simulink subsystem "SubsistemaMotor"  (R2022b)
settings: Solver=VariableStepAuto  StartTime=0.0  StopTime=10.0  RelTol=1e-3
libraries: arduinolib x6, simulink x2
settings Model: Creator=manu_  LastModifiedBy=manu_

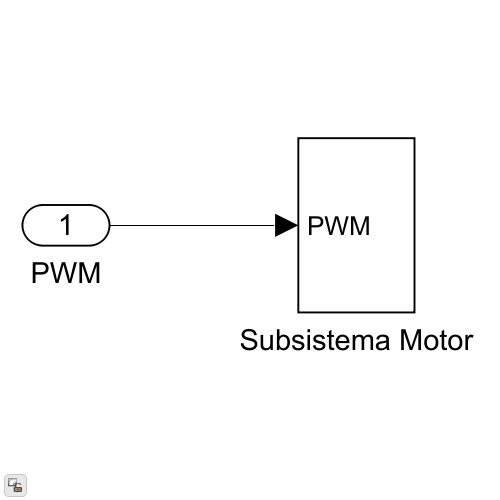
[thumbnail: Simulink's stored preview of the top-level diagram]
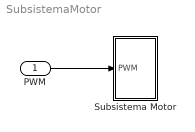
== system SubsistemaMotor ==
  PWM : Inport
  Subsistema Motor : Subsystem
  wires:
  PWM/1 -> Subsistema Motor/1(PWM)

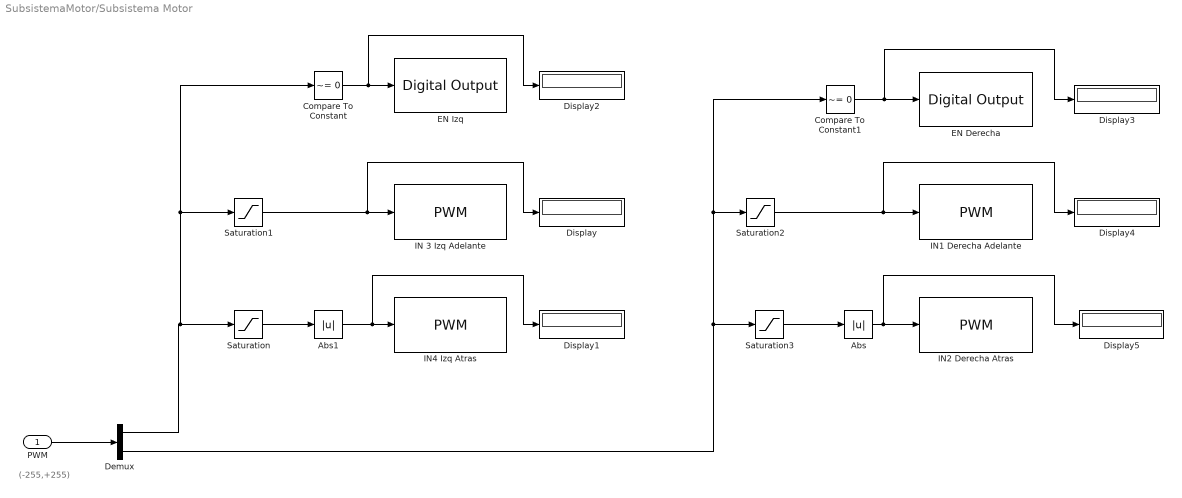
== system SubsistemaMotor/Subsistema Motor ==
  note: (-255,+255)
  PWM : Inport
  Abs : Abs  SaturateOnIntegerOverflow=off
  Abs1 : Abs  SaturateOnIntegerOverflow=off
  Compare To Constant : simulink/Logic and Bit Operations/Compare To Constant  relop=~=  const=0  OutDataTypeStr=boolean
  Compare To Constant1 : simulink/Logic and Bit Operations/Compare To Constant  relop=~=  const=0  OutDataTypeStr=boolean
  Demux : Demux  Outputs=2
  Display{,1..5} (6 alike) : Display
  EN Derecha : arduinolib/Digital Output  pinNumber=8  Direction=output  blockPlatform=arduino
  EN Izq : arduinolib/Digital Output  pinNumber=13  Direction=output  blockPlatform=arduino
  IN 3 Izq Adelante : arduinolib/PWM  pinNumber=11  frequencyType=Default  desiredFrequency=490.2  achievableFrequency=490.2
  IN1 Derecha Adelante : arduinolib/PWM  pinNumber=9  frequencyType=Default  desiredFrequency=490.2  achievableFrequency=490.2
  IN2 Derecha Atras : arduinolib/PWM  pinNumber=10  frequencyType=Default  desiredFrequency=490.2  achievableFrequency=490.2
  IN4 Izq Atras : arduinolib/PWM  pinNumber=12  frequencyType=Default  desiredFrequency=490.2  achievableFrequency=490.2
  Saturation : Saturate  UpperLimit=0  LowerLimit=-255
  Saturation1 : Saturate  UpperLimit=255  LowerLimit=1
  Saturation2 : Saturate  UpperLimit=255  LowerLimit=1
  Saturation3 : Saturate  UpperLimit=0  LowerLimit=-255
  wires:
  Saturation3/1 -> Abs/1
  Saturation/1 -> Abs1/1
  Saturation2/1 -> IN1 Derecha Adelante/1, Display4/1
  PWM/1 -> Demux/1
  Demux/1 -> Saturation/1, Saturation1/1, Compare To Constant/1
  Abs/1 -> IN2 Derecha Atras/1, Display5/1
  Demux/2 -> Saturation3/1, Saturation2/1, Compare To Constant1/1
  Saturation1/1 -> IN 3 Izq Adelante/1, Display/1
  Compare To Constant/1 -> EN Izq/1, Display2/1
  Compare To Constant1/1 -> EN Derecha/1, Display3/1
  Abs1/1 -> IN4 Izq Atras/1, Display1/1
